simulink model "HW03_Tirel_Sim2"  (R2020b)
settings: Solver=VariableStepAuto  StartTime=0.0  StopTime=20000  RelTol=1e-3
values from neighbouring files (symbols this model uses):
  Dec = tunableGain('Decoupler', eye(p))    [HW03_Tirel_Mat2.m]
  h1o = 16.3    [HW03_Tirel_Mat2.m]
  h2o = 13.7    [HW03_Tirel_Mat2.m]
undefined symbols (not defined in the file or in its folder): K2
libraries: cstblocks x5, pid_lib x2
settings Model: Creator=DELL  LastModifiedBy=DELL

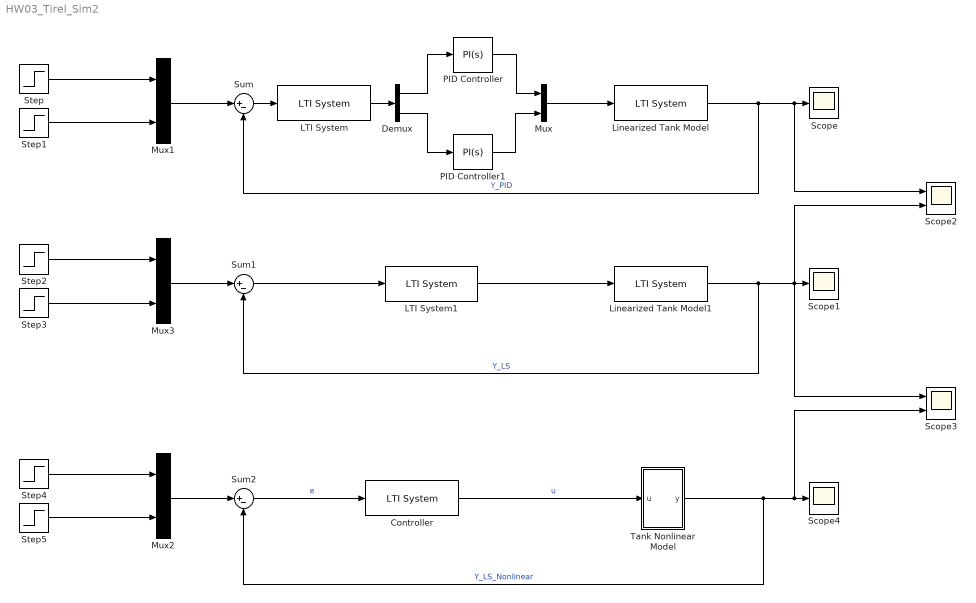
== system HW03_Tirel_Sim2 ==
  Controller : cstblocks/LTI System  sys=tf(K2)  IC=[]
  Demux : Demux  Outputs=2
  LTI System : cstblocks/LTI System  sys=tf(Dec)  IC=[]
  LTI System1 : cstblocks/LTI System  sys=tf(K2)  IC=[]
  Linearized Tank Model : cstblocks/LTI System  sys=W  IC=[]
  Linearized Tank Model1 : cstblocks/LTI System  sys=W  IC=[]
  Mux{,1..3} (4 alike) : Mux  Inputs=2
  PID Controller : pid_lib/PID Controller  Controller=PI  Form=Parallel  TimeDomain=Continuous-time  UseExternalTs=off  SampleTime=-1  IntegratorMethod=Forward Euler  FilterMethod=Forward Euler  ControllerParametersSource=internal  P=-0.0157  I=-1.9e-05  D=-17.5280408467088  UseFilter=on  N=0.0659216524889812  TunerSelectOption=Transfer Function Based (PID Tuner App)  InitialConditionSource=internal  InitialConditionForIntegrator=0  InitialConditionForFilter=0  DifferentiatorICPrevScaledInput=0  ExternalReset=none  TrackingMode=off  Kt=1  LimitOutput=off  SatLimitsSource=internal  UpperSaturationLimit=inf  LowerSaturationLimit=-inf  LinearizeAsGain=on  AntiWindupMode=none  Kb=1  POutMin=[]  POutMax=[]  IOutMin=[]  IOutMax=[]  DOutMin=[]  DOutMax=[]  NOutMin=[]  NOutMax=[]  SumOutMin=[]  SumOutMax=[]  SaturationOutMin=[]  SaturationOutMax=[]  PParamMin=[]  PParamMax=[]  IParamMin=[]  IParamMax=[]  DParamMin=[]  DParamMax=[]  NParamMin=[]  NParamMax=[]  KbParamMin=[]  KbParamMax=[]  KtParamMin=[]  KtParamMax=[]  KbOutMin=[]  KbOutMax=[]  KtOutMin=[]  KtOutMax=[]  IntegratorOutMin=[]  IntegratorOutMax=[]  FilterOutMin=[]  FilterOutMax=[]  SumI1OutMin=[]  SumI1OutMax=[]  SumI2OutMin=[]  SumI2OutMax=[]  SumI3OutMin=[]  SumI3OutMax=[]  SumI4OutMin=[]  SumI4OutMax=[]  SumDOutMin=[]  SumDOutMax=[]  DifferentiatorOutMin=[]  DifferentiatorOutMax=[]  FilterDiffOutCoefMin=[]  FilterDiffOutCoefMax=[]  ReciprocalOutMin=[]  ReciprocalOutMax=[]  SumDenOutMin=[]  SumDenOutMax=[]  SumNumOutMin=[]  SumNumOutMax=[]  DivideOutMin=[]  DivideOutMax=[]  UdiffTsProdOutMin=[]  UdiffTsProdOutMax=[]  NTsProdOutMin=[]  NTsProdOutMax=[]  UintegralTsProdOutMin=[]  UintegralTsProdOutMax=[]  UngainTsProdOutMin=[]  UngainTsProdOutMax=[]  IntegratorContinuousStateAttributes=''  IntegratorStateMustResolveToSignalObject=off  IntegratorRTWStateStorageClass=Auto  FilterContinuousStateAttributes=''  FilterStateMustResolveToSignalObject=off  FilterRTWStateStorageClass=Auto  ParallelPVariant=InternalParameters  IdealPVariant=Disabled  IVariant=InternalParameters  DVariant=Disabled  IntegratorVariant=Continuous  SatVariant=Disabled  AWVariant=Passthrough  PCopyVariant=Disabled  TRVariant=Disabled  FdbkBlocksVariant=Forward  IdealPFdbkVariant=Disabled  SatFdbkVariant=Disabled  DerivativeFilterVariant=Disabled  NVariant=Disabled  NCopyVariant=Disabled_SignalSpec  FilterICVariant=Disabled  IntegratorICVariant=InternalICs  ExternalResetVariant=Disabled  TRSumVariant=Passthrough  SumFdbkVariant=Disabled  SumVariant=Sum_PI  TsampFilterVariant=InternalTs  TsampNgainVariant=Passthrough  TsampIntegralVariant=Passthrough  ExternalSaturationOutDataTypeStr=Inherit: Same as second input
  PID Controller1 : pid_lib/PID Controller  Controller=PI  Form=Parallel  TimeDomain=Continuous-time  UseExternalTs=off  SampleTime=-1  IntegratorMethod=Forward Euler  FilterMethod=Forward Euler  ControllerParametersSource=internal  P=0.399  I=0.000556  D=-5.34576938199859  UseFilter=on  N=0.123252530997083  TunerSelectOption=Transfer Function Based (PID Tuner App)  InitialConditionSource=internal  InitialConditionForIntegrator=0  InitialConditionForFilter=0  DifferentiatorICPrevScaledInput=0  ExternalReset=none  TrackingMode=off  Kt=1  LimitOutput=off  SatLimitsSource=internal  UpperSaturationLimit=inf  LowerSaturationLimit=-inf  LinearizeAsGain=on  AntiWindupMode=none  Kb=1  POutMin=[]  POutMax=[]  IOutMin=[]  IOutMax=[]  DOutMin=[]  DOutMax=[]  NOutMin=[]  NOutMax=[]  SumOutMin=[]  SumOutMax=[]  SaturationOutMin=[]  SaturationOutMax=[]  PParamMin=[]  PParamMax=[]  IParamMin=[]  IParamMax=[]  DParamMin=[]  DParamMax=[]  NParamMin=[]  NParamMax=[]  KbParamMin=[]  KbParamMax=[]  KtParamMin=[]  KtParamMax=[]  KbOutMin=[]  KbOutMax=[]  KtOutMin=[]  KtOutMax=[]  IntegratorOutMin=[]  IntegratorOutMax=[]  FilterOutMin=[]  FilterOutMax=[]  SumI1OutMin=[]  SumI1OutMax=[]  SumI2OutMin=[]  SumI2OutMax=[]  SumI3OutMin=[]  SumI3OutMax=[]  SumI4OutMin=[]  SumI4OutMax=[]  SumDOutMin=[]  SumDOutMax=[]  DifferentiatorOutMin=[]  DifferentiatorOutMax=[]  FilterDiffOutCoefMin=[]  FilterDiffOutCoefMax=[]  ReciprocalOutMin=[]  ReciprocalOutMax=[]  SumDenOutMin=[]  SumDenOutMax=[]  SumNumOutMin=[]  SumNumOutMax=[]  DivideOutMin=[]  DivideOutMax=[]  UdiffTsProdOutMin=[]  UdiffTsProdOutMax=[]  NTsProdOutMin=[]  NTsProdOutMax=[]  UintegralTsProdOutMin=[]  UintegralTsProdOutMax=[]  UngainTsProdOutMin=[]  UngainTsProdOutMax=[]  IntegratorContinuousStateAttributes=''  IntegratorStateMustResolveToSignalObject=off  IntegratorRTWStateStorageClass=Auto  FilterContinuousStateAttributes=''  FilterStateMustResolveToSignalObject=off  FilterRTWStateStorageClass=Auto  ParallelPVariant=InternalParameters  IdealPVariant=Disabled  IVariant=InternalParameters  DVariant=Disabled  IntegratorVariant=Continuous  SatVariant=Disabled  AWVariant=Passthrough  PCopyVariant=Disabled  TRVariant=Disabled  FdbkBlocksVariant=Forward  IdealPFdbkVariant=Disabled  SatFdbkVariant=Disabled  DerivativeFilterVariant=Disabled  NVariant=Disabled  NCopyVariant=Disabled_SignalSpec  FilterICVariant=Disabled  IntegratorICVariant=InternalICs  ExternalResetVariant=Disabled  TRSumVariant=Passthrough  SumFdbkVariant=Disabled  SumVariant=Sum_PI  TsampFilterVariant=InternalTs  TsampNgainVariant=Passthrough  TsampIntegralVariant=Passthrough  ExternalSaturationOutDataTypeStr=Inherit: Same as second input
  Scope : Scope
  Scope1 : Scope
  Scope2 : Scope  NumInputPorts=2
  Scope3 : Scope  NumInputPorts=2
  Scope4 : Scope
  Step : Step  Time=0  After=h1o  SampleTime=0
  Step1 : Step  Time=0  After=h2o  SampleTime=0
  Step2 : Step  Time=0  After=h1o  SampleTime=0
  Step3 : Step  Time=0  After=h2o  SampleTime=0
  Step4 : Step  Time=0  After=h1o  SampleTime=0
  Step5 : Step  Time=0  After=h2o  SampleTime=0
  Sum : Sum  Inputs=|+-
  Sum1 : Sum  Inputs=|+-
  Sum2 : Sum  Inputs=|+-
  Tank Nonlinear Model : Subsystem
  wires:
  Sum/1 -> LTI System/1
  PID Controller/1 -> Mux/1
  PID Controller1/1 -> Mux/2
  Mux/1 -> Linearized Tank Model/1
  Linearized Tank Model/1 -> Scope2/1, Scope/1, Sum/2  "Y_PID"
  Step1/1 -> Mux1/2
  Step/1 -> Mux1/1
  Mux1/1 -> Sum/1
  LTI System/1 -> Demux/1
  Demux/1 -> PID Controller/1
  Demux/2 -> PID Controller1/1
  Step3/1 -> Mux3/2
  Mux3/1 -> Sum1/1
  Sum1/1 -> LTI System1/1
  Linearized Tank Model1/1 -> Scope2/2, Scope1/1, Scope3/1, Sum1/2  "Y_LS"
  Step2/1 -> Mux3/1
  LTI System1/1 -> Linearized Tank Model1/1
  Step4/1 -> Mux2/1
  Mux2/1 -> Sum2/1
  Step5/1 -> Mux2/2
  Sum2/1 -> Controller/1  "e"
  Tank Nonlinear Model/1(y) -> Scope3/2, Scope4/1, Sum2/2  "Y_LS_Nonlinear"
  Controller/1 -> Tank Nonlinear Model/1(u)  "u"

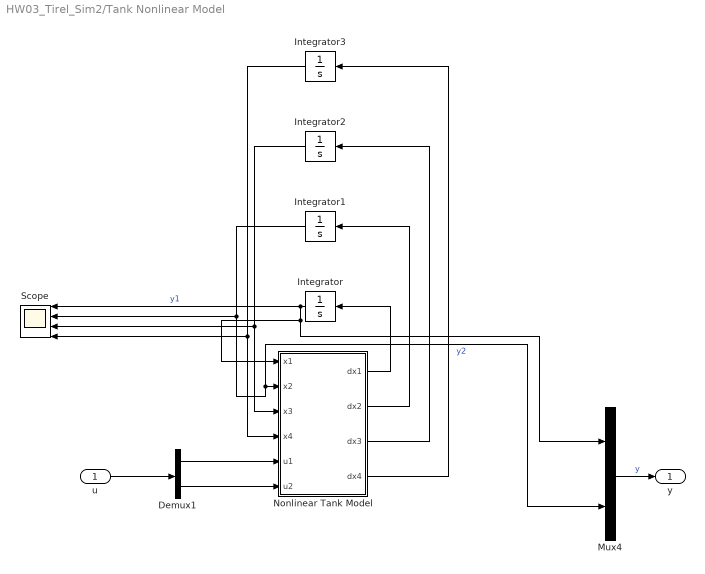
== system HW03_Tirel_Sim2/Tank Nonlinear Model ==
  u : Inport
  Demux1 : Demux  Outputs=2
  Integrator{,1..3} (4 alike) : Integrator
  Mux4 : Mux  Inputs=2
  Nonlinear Tank Model : MATLAB Function  TreatAsAtomicUnit=on
  Scope : Scope  NumInputPorts=4
  y : Outport
  wires:
  Demux1/2 -> Nonlinear Tank Model/6(u2)
  Integrator3/1 -> Scope/4, Nonlinear Tank Model/4(x4)
  Nonlinear Tank Model/3(dx3) -> Integrator2/1
  Nonlinear Tank Model/2(dx2) -> Integrator1/1
  Integrator/1 -> Scope/1, Mux4/1, Nonlinear Tank Model/1(x1)  "y1"
  Integrator1/1 -> Scope/2, Mux4/2, Nonlinear Tank Model/2(x2)  "y2"
  Demux1/1 -> Nonlinear Tank Model/5(u1)
  Integrator2/1 -> Scope/3, Nonlinear Tank Model/3(x3)
  u/1 -> Demux1/1
  Nonlinear Tank Model/4(dx4) -> Integrator3/1
  Nonlinear Tank Model/1(dx1) -> Integrator/1
  Mux4/1 -> y/1  "y"

== matlab function HW03_Tirel_Sim2/Tank Nonlinear Model/Nonlinear Tank Model ==
  data: x1 input; dx1 output; x2 input; x3 input; x4 input; u1 input; dx2 output; dx3 output; dx4 output; u2 input
function [dx1,dx2,dx3,dx4] = fcn(x1,x2,x3,x4,u1,u2)

g = 9.81; % m/s^2

% Nominal Levels of height of waters in the Tanks
h1o = 16.3; %cm 
h2o = 13.7; %cm 
h3o = 6.0; %cm 
h4o = 8.1; %cm 

% Ratio of flow 1-4 
gam1 = 0.3;
% Ratio of flow 2-3
gam2 = 0.3;

% Tank Area
A1 = 730; % cm^2
A2 = 730; % cm^2
A3 = 730; % cm^2
A4 = 730; % cm^2

% Drain Area
a1 = 2.05; % cm^2
a2 = 2.26; % cm^2
a3 = 2.37; % cm^2
a4 = 2.07; % cm^2

% Pumps Proportionallity Constants
k1 = 7.45; % cm^3/s %
k2 = 7.30; % cm^3/s %


dx1 = -(a1/A1)*sqrt(2*g*x1) + (a3/A1)*sqrt(2*g*x3) + (gam1*k1/A1)*u1;
dx2 = -(a2/A2)*sqrt(2*g*x2) + (a4/A2)*sqrt(2*g*x4) + (gam2*k2/A2)*u2;
dx3 = -(a3/A3)*sqrt(2*g*x3) + ((1-gam2)*k2/A3)*u2;
dx4 = -(a4/A4)*sqrt(2*g*x3) + ((1-gam1)*k1/A4)*u1;
